simulink library "levitron_lib"  (Simulink 7.1)
libraries: simulink x2
settings Model: Creator=volgy  LastModifiedBy=volgy

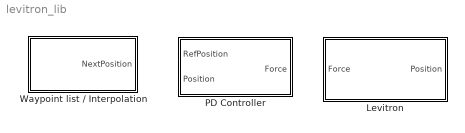
== system levitron_lib ==
  Levitron : Subsystem  mask{mass=1, gravity=-9.81, v0=15, z0=10}
      mask prompts: mass "Mass (g)"; gravity "Gravity (m/s^2)"; v0 "Initial velocity (m/s)"; z0 "Initial position (m)"
  PD Controller : Subsystem  mask{gain_p=6, gain_d=-5, gain=10, f_limit=100}
      mask prompts: gain_p "Proportional Gain"; gain_d "Difference Gain"; gain "Controller Gain"; f_limit "Controller Limit"
  Waypoint list / Interpolation : Subsystem  mask{sample_time=0.2, time_values=[0 20 40 60 80 100], output_values=[10 50 30 20 40 10]}
      mask prompts: sample_time "Sample Time (s)"; time_values "Time Values"; output_values "Output Values"

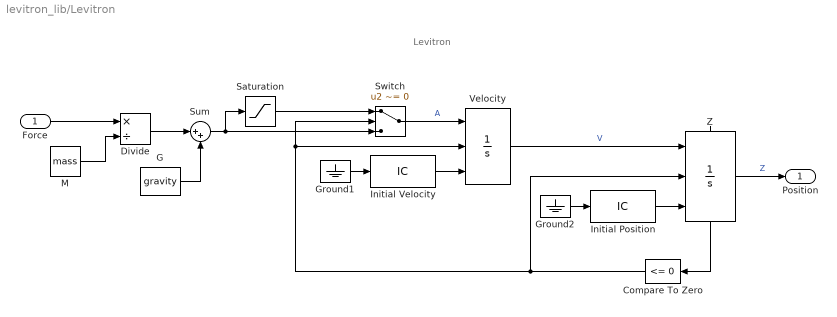
== system levitron_lib/Levitron ==
  note: Levitron
  Force : Inport  OutDataType=sfix(16)  OutScaling=2^0
  Compare To Zero : simulink/Logic and Bit Operations/Compare To Zero  Orientation=left  SystemSampleTime=-1  relop=<=  LogicOutDataTypeMode=boolean
  Divide : Product  Inputs=*/  OutDataType=sfix(16)  OutScaling=2^-10
  G : Constant  Value=gravity  OutDataType=sfix(16)  OutScaling=2^0
  Ground1 : Ground
  Ground2 : Ground
  Initial Position : InitialCondition  Value=z0
  Initial Velocity : InitialCondition  Value=v0
  M : Constant  Value=mass  OutDataType=sfix(16)  OutScaling=2^0
  Saturation : Saturate  UpperLimit=inf  LowerLimit=0.0  OutDataType=sfix(16)  OutScaling=2^0
  Sum : Sum  Inputs=|++  OutDataType=sfix(16)  OutScaling=2^0
  Switch : Switch  Criteria=u2 ~= 0  OutDataType=sfix(16)  OutScaling=2^0
  Velocity : Integrator  ExternalReset=rising  InitialConditionSource=external
  Z : Integrator  ExternalReset=rising  InitialConditionSource=external  InitialCondition=10  LimitOutput=on  LowerSaturationLimit=0  ShowStatePort=on
      settings: AttributesFormatString=Xo = %<InitialCondition>
  Position : Outport  OutDataType=sfix(16)  OutScaling=2^0
  wires:
  Force/1 -> Divide/1
  Z/1 -> Position/1  "Z"
  G/1 -> Sum/2
  Divide/1 -> Sum/1
  M/1 -> Divide/2
  Sum/1 -> Saturation/1, Switch/3
  Saturation/1 -> Switch/1
  Switch/1 -> Velocity/1  "A"
  Ground1/1 -> Initial Velocity/1
  Z/State -> Compare To Zero/1
  Initial Position/1 -> Z/3
  Compare To Zero/1 -> Velocity/2, Switch/2, Z/2
  Ground2/1 -> Initial Position/1
  Velocity/1 -> Z/1  "V"
  Initial Velocity/1 -> Velocity/3

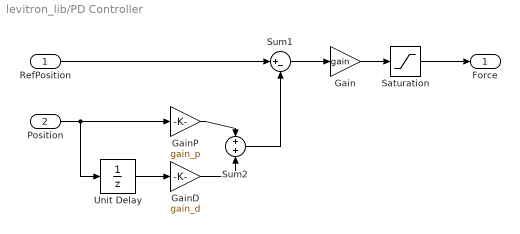
== system levitron_lib/PD Controller ==
  RefPosition : Inport
  Position : Inport  Port=2
  Gain : Gain  Gain=gain  ParameterDataType=sfix(16)  ParameterScaling=2^0  OutDataType=sfix(16)  OutScaling=2^0
  GainD : Gain  Gain=gain_d  ParameterDataType=sfix(16)  ParameterScaling=2^0  OutDataType=sfix(16)  OutScaling=2^0
  GainP : Gain  Gain=gain_p  ParameterDataType=sfix(16)  ParameterScaling=2^0  OutDataType=sfix(16)  OutScaling=2^0
  Saturation : Saturate  UpperLimit=f_limit  LowerLimit=0  OutDataType=sfix(16)  OutScaling=2^0
  Sum1 : Sum  Inputs=|+-  OutDataType=sfix(16)  OutScaling=2^0
  Sum2 : Sum  Inputs=+|+  OutDataType=sfix(16)  OutScaling=2^0
  Unit Delay : UnitDelay  X0=10  SampleTime=-1
  Force : Outport
  wires:
  Sum2/1 -> Sum1/2
  Position/1 -> Unit Delay/1, GainP/1
  RefPosition/1 -> Sum1/1
  Saturation/1 -> Force/1
  Gain/1 -> Saturation/1
  Sum1/1 -> Gain/1
  GainD/1 -> Sum2/2
  GainP/1 -> Sum2/1
  Unit Delay/1 -> GainD/1

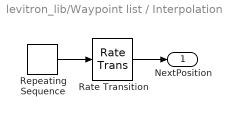
== system levitron_lib/Waypoint list / Interpolation ==
  Rate Transition : RateTransition  OutPortSampleTime=sample_time
  Repeating Sequence : simulink/Sources/Repeating Sequence  SystemSampleTime=-1  rep_seq_t=time_values  rep_seq_y=output_values
  NextPosition : Outport
  wires:
  Repeating Sequence/1 -> Rate Transition/1
  Rate Transition/1 -> NextPosition/1
